simulink model "Aircraft_Power_Network"  (R2020a)
settings: Solver=ode23t  StartTime=0.0  StopTime=40  RelTol=1e-3  EnableMultiTasking=on
PostLoadFcn:
  | %load PQ_DATA4
  | Flight_Cycle_Num = 1;
  | 
  | warning off Simulink:blocks:MatchingFromNotFound
  | warning off Simulink:blocks:MatchingGotoNotFound
  | warning off Simulink:Engine:SaveWithParameterizedLinks_Warning
  | warning off MATLAB:nearlySingularMatrix
  | warning off simscape:compiler:sli:init:SolverNotRecommended
  | warning off Simulink:ID:DuplicateSID
  | warning off Simulink:Engine:UINotUpdatedDuringRapidAccelSim
  | warning off Simulink:SampleTime:IllegalIPortRateTrans
  | warning off Simulink:SampleTime:SourceInheritedTS
StartFcn:
  | tic;
StopFcn:
  | Elapsed_Sim_Time = toc; disp(['Elapsed time is ' num2str(Elapsed_Sim_Time)])
undefined symbols (not defined in the file or in its folder): Ts
libraries: powerlib x6, powerlib_meascontrol x4, Actuator_AC_Lib x2, Lamp_Lib x2, Pump_Lib x2, DC_Loads_Lib x2, Distribution_Lib x1, Generator_Lib x1, Power_Calc_Lib x1
Description:
  | Copyright 2014-2020 The MathWorks, Inc.
settings Model: TunableVars=Flight_Cycle_Num  TunableVarsStorageClass=Auto  Creator=smiller  LastModifiedBy=smiller
settings DataIOCC: LimitDataPoints=on  SaveFormat=Array  ReturnWorkspaceOutputs=off
settings OptimizationCC: DefaultParameterBehavior=Inlined  OptimizeBlockIOStorage=off  BufferReuse=off  GlobalBufferReuse=off  ExpressionFolding=off  LocalBlockOutputs=off  LifeSpan=inf  OptimizeDataStoreBuffers=off  BusAssignmentInplaceUpdate=off
settings DebuggingCC: UnderspecifiedInitializationDetection=Classic  MergeDetectMultiDrivingBlocksExec=none  SolverPrmCheckMsg=warning  MultiTaskRateTransMsg=warning  AllowSymbolicDim=off  StateNameClashWarn=warning  PregeneratedLibrarySubsystemCodeDiagnostic=none  SFUnexpectedBacktrackingDiag=warning  SFNoUnconditionalDefaultTransitionDiag=warning  SFExecutionAtInitializationDiag=none  ArithmeticOperatorsInVariantConditions=warning
settings HardwareCC: ProdBitPerPointer=32  ProdBitPerSizeT=32  ProdBitPerPtrDiffT=32  ProdLargestAtomicFloat=None  ProdIntDivRoundTo=Undefined  ProdEndianess=Unspecified  ProdWordSize=32  ProdHWDeviceType=32-bit Generic
settings ModelReferenceCC: PropagateSignalLabelsOutOfModel=off
settings SFSimCC: SimUseLocalCustomCode=off  CustomCodeUndefinedFunction=UseInterfaceOnly
settings RTWCC: RTWUseLocalCustomCode=off
settings CodeAppCC: StateflowObjectComments=on
settings GRTTargetCC: TargetLangStandard=C89/C90 (ANSI)  CombineOutputUpdateFcns=off  GRTInterface=on
settings ConfigComp: CovMetricSettings=dw  CovHtmlReporting=on  CovSaveCumulativeToWorkspaceVar=on  CovSaveSingleToWorkspaceVar=on  CovExternalEMLEnable=off  CovSFcnEnable=off
settings SimscapeCC: SimscapeNormalizeSystem=off

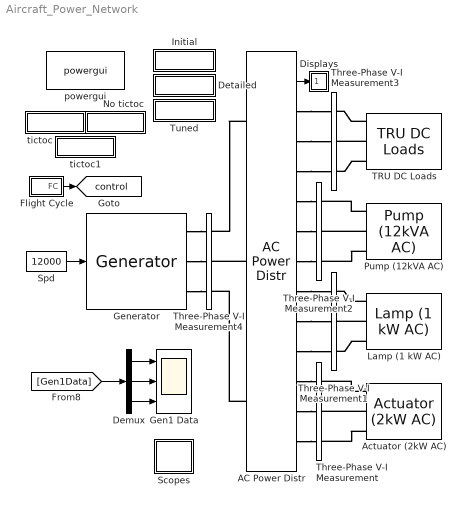
== system Aircraft_Power_Network ==
  AC Power Distr : Distribution_Lib/AC Power Distr  LabelModeActiveChoice=Phasor  ModelType=Phasor
      settings: AttributesFormatString=%<BlockChoice>
  Actuator (2kW AC) : Actuator_AC_Lib/Actuator (2kW AC)  LabelModeActiveChoice=Phasor  ModelType=Phasor  PQ_Model=Tuned
      link override Detailed/PM Synchronous Motor Drive/Output Bus Selector: OutputSignals=Rotor speed wm (rad/s)
      link override Detailed/PM Synchronous Motor Drive/Permanent Magnet Synchronous Machine: MechanicalLoad=Torque Tm  VoltageCst=126.966  TorqueCst=1.05
      link override Detailed/PM Synchronous Motor Drive/VECT: modulationType=Hysteresis  Ts_vect=20e-6  h=0.1  freq_max=20e3  fc_bus=50  car_freq=20000  nb_p=4  machineConstant=Flux linkage established by magnets (V.s)  fluxConstant=0.175  voltageConstant=126.966  torqueConstant=1.05  kp_Id=200  ki_Id=1000  kp_Iq=200  ki_Iq=1000
      link override Detailed/PM Synchronous Motor Drive1/VECT: freq_max=20e3  Ts_vect=50e-6  h=0.1  nb_p=4  lambda=0.175
      link override Phasor/Calc PQ: BlockChoice=Initial
      settings: AttributesFormatString=%<BlockChoice>
  Demux : Demux  Outputs=[2 1 1]
  Detailed : Subsystem
      settings: OpenFcn=Select_APN_Model_Config(bdroot,'Detailed');
      mask Display: disp('Detailed');
  Displays : Subsystem
      mask Display: disp('D')
  Flight Cycle : Subsystem
      mask Display: disp(num2str(evalin('base','Flight_Cycle_Num')));
  Gen1 Data : Scope  NumInputPorts=3
  Generator : Generator_Lib/Generator  LabelModeActiveChoice=Ideal  GenType=Ideal  GenTypeDCLink=Ideal
      link override VSCF DC Link/DC Link Gen: BlockChoice=Ideal
      link override VSCF DC Link/DC Link Gen/Sync Mach/Simplified Synchronous Machine SI Units/Electrical model: BlockChoice=Phasor
      link override VSCF DC Link/DC Link Gen/Sync Mach/Simplified Synchronous Machine SI Units/From: GotoTag=tp2df5cfb3_b42e_4dd4_aed6_ebb45f5ee09b
      link override VSCF DC Link/DC Link Gen/Sync Mach/Simplified Synchronous Machine SI Units/Goto: GotoTag=tp9f3ab3a0_63ac_4acf_b3bd_c670964be41e
      link override VSCF DC Link/DC Link Gen/Sync Mach/Simplified Synchronous Machine SI Units/Mechanical model: BlockChoice=Phasor w input
      settings: AttributesFormatString=%<BlockChoice>
  Initial : Subsystem
      settings: OpenFcn=Select_APN_Model_Config(bdroot,'Initial');
      mask Display: disp('Initial');
  Lamp (1 kW AC) : Lamp_Lib/Lamp (1 kW AC)  RequirementInfo={} %GIDa_b4ebd6a2_cdd2_4eca_9ae5_96943b3eee14  LabelModeActiveChoice=Phasor  ModelType=Phasor  PQ_Model=Tuned
      link override Phasor/Calc PQ: BlockChoice=Initial
      settings: AttributesFormatString=%<BlockChoice>
  No tictoc : Subsystem
      settings: OpenFcn=|
      | set_param(bdroot,'StartFcn','');
      | set_param(bdroot,'StopFcn','');
      mask Display: disp('No tictoc')
  Pump (12kVA AC) : Pump_Lib/Pump (12kVA AC)  LabelModeActiveChoice=Phasor  ModelType=Phasor  PQ_Model=Tuned
      link override Phasor/Calc PQ: BlockChoice=Initial
      settings: AttributesFormatString=%<BlockChoice>
  Scopes : Subsystem
  Spd : Constant  Value=12000
  TRU DC Loads : DC_Loads_Lib/TRU DC Loads  RequirementInfo={} %GIDa_0f590c74_ec2b_4e2c_b0ce_7c36d608bdaa  LabelModeActiveChoice=Phasor  ModelType=Phasor  PQ_Model=Tuned
      link override Phasor/Calc PQ: BlockChoice=Initial
      settings: AttributesFormatString=%<BlockChoice>
  Three-Phase V-I Measurement : powerlib/Measurements/Three-Phase V-I Measurement  VoltageMeasurement=phase-to-ground  SetLabelV=on  LabelV=Vabc_BDMotor  Vpu=off  VpuLL=off  CurrentMeasurement=yes  SetLabelI=on  LabelI=Iabc_BDMotor  Ipu=off  Pbase=100e6  Vbase=500e3  OutputType=Magnitude  PhasorSimulation=on  PSBequivalent=0
  Three-Phase V-I Measurement1 : powerlib/Measurements/Three-Phase V-I Measurement  VoltageMeasurement=phase-to-ground  SetLabelV=on  LabelV=Vabc_Lamp  Vpu=off  VpuLL=off  CurrentMeasurement=yes  SetLabelI=on  LabelI=Iabc_Lamp  Ipu=off  Pbase=100e6  Vbase=500e3  OutputType=Magnitude  PhasorSimulation=on  PSBequivalent=0
  Three-Phase V-I Measurement2 : powerlib/Measurements/Three-Phase V-I Measurement  VoltageMeasurement=phase-to-ground  SetLabelV=on  LabelV=Vabc_InductionMotor  Vpu=off  VpuLL=off  CurrentMeasurement=yes  SetLabelI=on  LabelI=Iabc_InductionMotor  Ipu=off  Pbase=100e6  Vbase=500e3  OutputType=Magnitude  PhasorSimulation=on  PSBequivalent=0
  Three-Phase V-I Measurement3 : powerlib/Measurements/Three-Phase V-I Measurement  VoltageMeasurement=phase-to-ground  SetLabelV=on  LabelV=Vabc_TRU  Vpu=off  VpuLL=off  CurrentMeasurement=yes  SetLabelI=on  LabelI=Iabc_TRU  Ipu=off  Pbase=100e6  Vbase=500e3  OutputType=Magnitude  PhasorSimulation=on  PSBequivalent=0
  Three-Phase V-I Measurement4 : powerlib/Measurements/Three-Phase V-I Measurement  VoltageMeasurement=phase-to-ground  SetLabelV=on  LabelV=Vabc_GEN  Vpu=off  VpuLL=off  CurrentMeasurement=yes  SetLabelI=on  LabelI=Iabc_GEN  Ipu=off  Pbase=100e6  Vbase=500e3  OutputType=Magnitude  PhasorSimulation=on  PSBequivalent=0
  Tuned : Subsystem
      settings: OpenFcn=Select_APN_Model_Config(bdroot,'Tuned');
      mask Display: disp('Tuned');
  powergui : powerlib/powergui  SimulationMode=Phasor  SampleTime=Ts  frequency=400  Iterations=50  frequencyindice=400  Pbase=100e6  ErrMax=0.0001  UnitsV=kV  UnitsW=MW  buscounter=0  FunctionMessages=off  echomessages=off  EnableUseOfTLC=off  CurrentSourceSwitches=off  DisableSnubberDevices=off  DisableRonSwitches=off  DisableVfSwitches=off  DisplayEquations=off  AutomaticDiscreteSolvers=off  SolverType=Tustin  Interpol=off  ExternalGateDelay=off  methode=off  Ts=0  x0status=blocks  SPID=off  SwTol=0  HookPort=off  NonlinearTolerance=0  nMaxIteration=15  ContinueOnMaxIteration=off  RestoreLinks=no  ResistiveCurrentMeasurement=off  Frange=[0:2:500]  Ylog=off  Xlog=on  ShowGrid=off  save=off  variable=ZData  structure=Gen1_Vab  ZoomFFT=on  StartTime=0.3  cycles=1  DisplayStyle=1  fundamental=400  FreqAxis=on  MaxFrequency=8000  frequencyindicesteady=1  RmsSteady=1  display=off
  tictoc : Subsystem
      settings: OpenFcn=|
      | set_param(bdroot,'StartFcn','tic;');
      | set_param(bdroot,'StopFcn','Elapsed_Sim_Time = toc; disp([''Elapsed time is '' num2str(Elapsed_Sim_Time)])');
      mask Display: disp('tictoc')
  tictoc1 : Subsystem
      settings: OpenFcn=open('APN_Demo_Script.html')
      mask Display: disp('Script')
  tag scope: control=global
  wires:
  Flight Cycle/1(FC) -> [control]
  AC Power Distr/1 -> Displays/1(In1)
  Spd/1 -> Generator/1
  [Gen1Data] -> Demux/1
  Demux/1 -> Gen1 Data/1
  Demux/2 -> Gen1 Data/2
  Demux/3 -> Gen1 Data/3
  connections:
  Generator/RConn1 -- Three-Phase V-I Measurement4/LConn1
  Generator/RConn2 -- Three-Phase V-I Measurement4/LConn2
  Generator/RConn3 -- Three-Phase V-I Measurement4/LConn3
  AC Power Distr/LConn2 -- Three-Phase V-I Measurement4/RConn2
  Lamp (1 kW AC)/LConn3 -- Three-Phase V-I Measurement1/RConn3
  Actuator (2kW AC)/LConn2 -- Three-Phase V-I Measurement/RConn2
  AC Power Distr/RConn3 -- Three-Phase V-I Measurement3/LConn3
  AC Power Distr/RConn6 -- Three-Phase V-I Measurement2/LConn3
  Pump (12kVA AC)/LConn2 -- Three-Phase V-I Measurement2/RConn2
  TRU DC Loads/LConn3 -- Three-Phase V-I Measurement3/RConn3
  Actuator (2kW AC)/LConn3 -- Three-Phase V-I Measurement/RConn3
  Pump (12kVA AC)/LConn3 -- Three-Phase V-I Measurement2/RConn3
  AC Power Distr/RConn4 -- Three-Phase V-I Measurement2/LConn1
  TRU DC Loads/LConn1 -- Three-Phase V-I Measurement3/RConn1
  AC Power Distr/RConn11 -- Three-Phase V-I Measurement/LConn2
  Actuator (2kW AC)/LConn1 -- Three-Phase V-I Measurement/RConn1
  AC Power Distr/RConn8 -- Three-Phase V-I Measurement1/LConn2
  AC Power Distr/LConn3 -- Three-Phase V-I Measurement4/RConn3
  AC Power Distr/LConn1 -- Three-Phase V-I Measurement4/RConn1
  AC Power Distr/RConn12 -- Three-Phase V-I Measurement/LConn3
  AC Power Distr/RConn1 -- Three-Phase V-I Measurement3/LConn1
  AC Power Distr/RConn5 -- Three-Phase V-I Measurement2/LConn2
  AC Power Distr/RConn9 -- Three-Phase V-I Measurement1/LConn3
  TRU DC Loads/LConn2 -- Three-Phase V-I Measurement3/RConn2
  AC Power Distr/RConn7 -- Three-Phase V-I Measurement1/LConn1
  Lamp (1 kW AC)/LConn2 -- Three-Phase V-I Measurement1/RConn2
  AC Power Distr/RConn10 -- Three-Phase V-I Measurement/LConn1
  Lamp (1 kW AC)/LConn1 -- Three-Phase V-I Measurement1/RConn1
  AC Power Distr/RConn2 -- Three-Phase V-I Measurement3/LConn2
  Pump (12kVA AC)/LConn1 -- Three-Phase V-I Measurement2/RConn1

== system Aircraft_Power_Network/Detailed ==

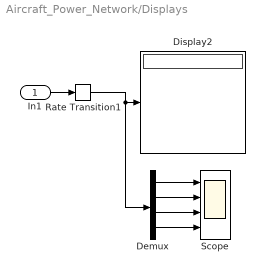
== system Aircraft_Power_Network/Displays ==
  In1 : Inport
  Demux : Demux
  Display2 : Display
      settings: Decimation=100  SampleTime=1e-2
  Rate Transition1 : RateTransition  OutPortSampleTimeOpt=Inherit  OutPortSampleTime=Ts
  Scope : Scope  NumInputPorts=4
  wires:
  In1/1 -> Rate Transition1/1
  Rate Transition1/1 -> Demux/1, Display2/1
  Demux/3 -> Scope/3
  Demux/4 -> Scope/4
  Demux/1 -> Scope/1
  Demux/2 -> Scope/2

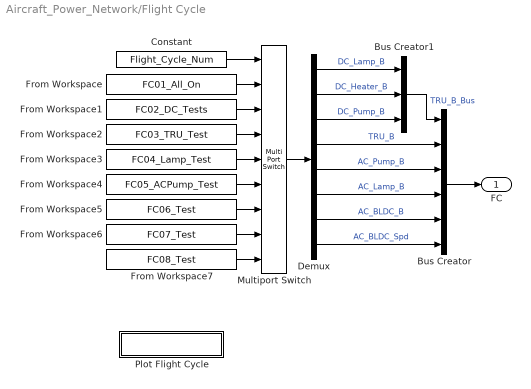
== system Aircraft_Power_Network/Flight Cycle ==
  Bus Creator : BusCreator  Inputs=6
  Bus Creator1 : BusCreator  Inputs=3
  Constant : Constant  Value=Flight_Cycle_Num
  Demux : Demux  Outputs=8
  From Workspace : FromWorkspace  VariableName=FC01_All_On  OutputAfterFinalValue=Holding final value
  From Workspace1 : FromWorkspace  VariableName=FC02_DC_Tests
  From Workspace2 : FromWorkspace  VariableName=FC03_TRU_Test
  From Workspace3 : FromWorkspace  VariableName=FC04_Lamp_Test
  From Workspace4 : FromWorkspace  VariableName=FC05_ACPump_Test  OutputAfterFinalValue=Holding final value
  From Workspace5 : FromWorkspace  VariableName=FC06_Test  OutputAfterFinalValue=Holding final value
  From Workspace6 : FromWorkspace  VariableName=FC07_Test  OutputAfterFinalValue=Holding final value
  From Workspace7 : FromWorkspace  VariableName=FC08_Test  OutputAfterFinalValue=Holding final value
  Multiport Switch : MultiPortSwitch  Inputs=8
  Plot Flight Cycle : Subsystem
      settings: OpenFcn=Plot_FC
      mask Display: disp('Plot Flight Cycle');
  FC : Outport  VectorParamsAs1DForOutWhenUnconnected=off
  wires:
  Bus Creator/1 -> FC/1
  Bus Creator1/1 -> Bus Creator/1  "TRU_B_Bus"
  From Workspace/1 -> Multiport Switch/2
  From Workspace1/1 -> Multiport Switch/3
  From Workspace2/1 -> Multiport Switch/4
  From Workspace3/1 -> Multiport Switch/5
  From Workspace4/1 -> Multiport Switch/6
  Multiport Switch/1 -> Demux/1
  Constant/1 -> Multiport Switch/1
  Demux/1 -> Bus Creator1/1  "DC_Lamp_B"
  Demux/2 -> Bus Creator1/2  "DC_Heater_B"
  Demux/3 -> Bus Creator1/3  "DC_Pump_B"
  Demux/4 -> Bus Creator/2  "TRU_B"
  Demux/5 -> Bus Creator/3  "AC_Pump_B"
  Demux/6 -> Bus Creator/4  "AC_Lamp_B"
  Demux/7 -> Bus Creator/5  "AC_BLDC_B"
  Demux/8 -> Bus Creator/6  "AC_BLDC_Spd"
  From Workspace5/1 -> Multiport Switch/7
  From Workspace6/1 -> Multiport Switch/8
  From Workspace7/1 -> Multiport Switch/9

== system Aircraft_Power_Network/Initial ==

== system Aircraft_Power_Network/No tictoc ==

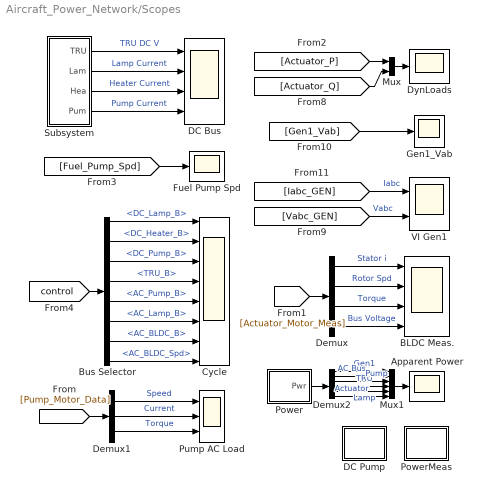
== system Aircraft_Power_Network/Scopes ==
  Apparent Power : Scope
  BLDC Meas. : Scope  NumInputPorts=4
  Bus Selector : BusSelector  OutputSignals=TRU_B_Bus.DC_Lamp_B,TRU_B_Bus.DC_Heater_B,TRU_B_Bus.DC_Pump_B,TRU_B,AC_Pump_B,AC_Lamp_B,AC_BLDC_B,AC_BLDC_Spd
  Cycle : Scope  NumInputPorts=8
  DC Bus : Scope  NumInputPorts=4
  DC Pump : Subsystem
  Demux : Demux  Outputs=[1 2 2 1]
  Demux1 : Demux  Outputs=3
  Demux2 : Demux  Outputs=6
  DynLoads : Scope
  Fuel Pump Spd : Scope
  Gen1_Vab : Scope
  Mux : Mux  Inputs=2
  Mux1 : Mux  Inputs=6
  Power : Subsystem
  PowerMeas : Subsystem
  Pump AC Load : Scope  NumInputPorts=3
  Subsystem : Subsystem
  VI Gen1 : Scope  NumInputPorts=2
  wires:
  [Fuel_Pump_Spd] -> Fuel Pump Spd/1
  Demux/1 -> BLDC Meas./1  "Stator i"
  Demux/2 -> BLDC Meas./2  "Rotor Spd"
  Demux/3 -> BLDC Meas./3  "Torque"
  Demux/4 -> BLDC Meas./4  "Bus Voltage"
  [Actuator_Motor_Meas] -> Demux/1
  Subsystem/2(Lam) -> DC Bus/2  "Lamp Current"
  Subsystem/3(Hea) -> DC Bus/3  "Heater Current"
  Subsystem/4(Pum) -> DC Bus/4  "Pump Current"
  Subsystem/1(TRU) -> DC Bus/1  "TRU DC V"
  [Gen1_Vab] -> Gen1_Vab/1
  [control] -> Bus Selector/1
  Bus Selector/8 -> Cycle/8  "<AC_BLDC_Spd>"
  Bus Selector/7 -> Cycle/7  "<AC_BLDC_B>"
  Bus Selector/5 -> Cycle/5  "<AC_Pump_B>"
  Bus Selector/6 -> Cycle/6  "<AC_Lamp_B>"
  Bus Selector/1 -> Cycle/1  "<DC_Lamp_B>"
  Bus Selector/2 -> Cycle/2  "<DC_Heater_B>"
  Bus Selector/4 -> Cycle/4  "<TRU_B>"
  Bus Selector/3 -> Cycle/3  "<DC_Pump_B>"
  [Actuator_P] -> Mux/1
  Mux/1 -> DynLoads/1
  [Actuator_Q] -> Mux/2
  [Iabc_GEN] -> VI Gen1/1  "Iabc"
  [Vabc_GEN] -> VI Gen1/2  "Vabc"
  Power/1(Pwr) -> Demux2/1
  Demux1/3 -> Pump AC Load/3  "Torque"
  Demux1/1 -> Pump AC Load/1  "Speed"
  Demux1/2 -> Pump AC Load/2  "Current"
  [Pump_Motor_Data] -> Demux1/1
  Demux2/6 -> Mux1/6  "Actuator"
  Demux2/1 -> Mux1/1  "Gen1"
  Demux2/2 -> Mux1/2  "AC Bus"
  Demux2/4 -> Mux1/4  "TRU"
  Demux2/3 -> Mux1/3  "Pump"
  Demux2/5 -> Mux1/5  "Lamp"
  Mux1/1 -> Apparent Power/1

== system Aircraft_Power_Network/Tuned ==

== system Aircraft_Power_Network/tictoc ==

== system Aircraft_Power_Network/tictoc1 ==

== system Aircraft_Power_Network/Flight Cycle/Plot Flight Cycle ==

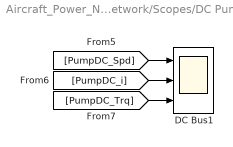
== system Aircraft_Power_Network/Scopes/DC Pump ==
  DC Bus1 : Scope  NumInputPorts=3
  wires:
  [PumpDC_i] -> DC Bus1/2
  [PumpDC_Spd] -> DC Bus1/1
  [PumpDC_Trq] -> DC Bus1/3

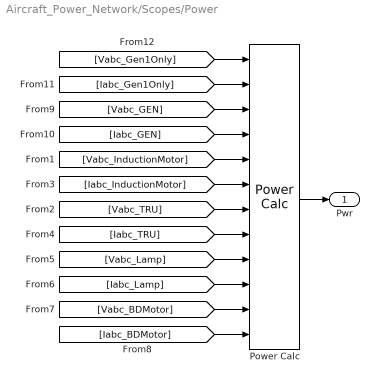
== system Aircraft_Power_Network/Scopes/Power ==
  Power Calc : Power_Calc_Lib/Power Calc  LabelModeActiveChoice=Phasor  ModelType=Phasor
      settings: AttributesFormatString=%<BlockChoice>
  Pwr : Outport  VectorParamsAs1DForOutWhenUnconnected=off
  wires:
  [Vabc_Gen1Only] -> Power Calc/1
  [Iabc_Gen1Only] -> Power Calc/2
  [Vabc_GEN] -> Power Calc/3
  [Iabc_GEN] -> Power Calc/4
  [Vabc_InductionMotor] -> Power Calc/5
  [Iabc_InductionMotor] -> Power Calc/6
  [Vabc_TRU] -> Power Calc/7
  [Iabc_TRU] -> Power Calc/8
  [Vabc_Lamp] -> Power Calc/9
  [Iabc_Lamp] -> Power Calc/10
  Power Calc/1 -> Pwr/1
  [Vabc_BDMotor] -> Power Calc/11
  [Iabc_BDMotor] -> Power Calc/12

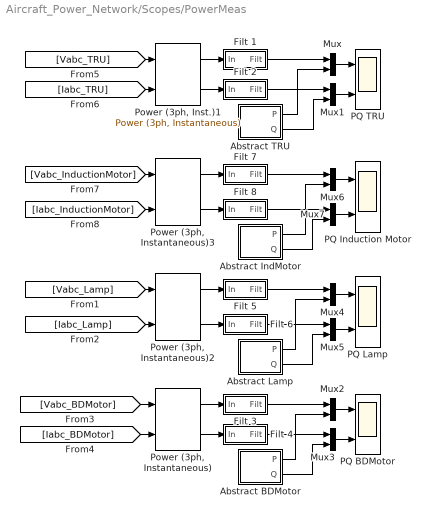
== system Aircraft_Power_Network/Scopes/PowerMeas ==
  Abstract BDMotor : Subsystem
  Abstract IndMotor : Subsystem
  Abstract Lamp : Subsystem
  Abstract TRU : Subsystem
  Filt 1 : Subsystem
  Filt 2 : Subsystem
  Filt 3 : Subsystem
  Filt 4 : Subsystem
  Filt 5 : Subsystem
  Filt 6 : Subsystem
  Filt 7 : Subsystem
  Filt 8 : Subsystem
  Mux{,1..7} (8 alike) : Mux  Inputs=2
  PQ BDMotor : Scope  NumInputPorts=2
  PQ Induction Motor : Scope  NumInputPorts=2
  PQ Lamp : Scope  NumInputPorts=2
  PQ TRU : Scope  NumInputPorts=2
  "Power (3ph, Instantaneous)" : powerlib_meascontrol/Measurements/Power (3ph, Instantaneous)
  "Power (3ph, Instantaneous)2" : powerlib_meascontrol/Measurements/Power (3ph, Instantaneous)
  "Power (3ph, Instantaneous)3" : powerlib_meascontrol/Measurements/Power (3ph, Instantaneous)
  "Power (3ph, Inst.)1" : powerlib_meascontrol/Measurements/Power (3ph, Instantaneous)
  wires:
  Filt 3/1(Filt) -> Mux2/1
  [Vabc_BDMotor] -> "Power (3ph, Instantaneous)"/1
  [Iabc_TRU] -> "Power (3ph, Inst.)1"/2
  Filt 1/1(Filt) -> Mux/1
  "Power (3ph, Inst.)1"/2 -> Filt 2/1(In)
  "Power (3ph, Instantaneous)"/1 -> Filt 3/1(In)
  [Iabc_BDMotor] -> "Power (3ph, Instantaneous)"/2
  "Power (3ph, Instantaneous)"/2 -> Filt 4/1(In)
  Filt 2/1(Filt) -> Mux1/1
  [Vabc_TRU] -> "Power (3ph, Inst.)1"/1
  "Power (3ph, Inst.)1"/1 -> Filt 1/1(In)
  Filt 4/1(Filt) -> Mux3/1
  [Iabc_Lamp] -> "Power (3ph, Instantaneous)2"/2
  "Power (3ph, Instantaneous)2"/2 -> Filt 6/1(In)
  [Vabc_Lamp] -> "Power (3ph, Instantaneous)2"/1
  "Power (3ph, Instantaneous)2"/1 -> Filt 5/1(In)
  [Iabc_InductionMotor] -> "Power (3ph, Instantaneous)3"/2
  Filt 7/1(Filt) -> Mux6/1
  "Power (3ph, Instantaneous)3"/2 -> Filt 8/1(In)
  Filt 8/1(Filt) -> Mux7/1
  [Vabc_InductionMotor] -> "Power (3ph, Instantaneous)3"/1
  "Power (3ph, Instantaneous)3"/1 -> Filt 7/1(In)
  Mux/1 -> PQ TRU/1
  Mux1/1 -> PQ TRU/2
  Mux2/1 -> PQ BDMotor/1
  Mux3/1 -> PQ BDMotor/2
  Filt 5/1(Filt) -> Mux4/1
  Filt 6/1(Filt) -> Mux5/1
  Mux4/1 -> PQ Lamp/1
  Mux5/1 -> PQ Lamp/2
  Abstract TRU/1(P) -> Mux/2
  Abstract TRU/2(Q) -> Mux1/2
  Abstract BDMotor/1(P) -> Mux2/2
  Abstract BDMotor/2(Q) -> Mux3/2
  Abstract Lamp/1(P) -> Mux4/2
  Abstract Lamp/2(Q) -> Mux5/2
  Mux6/1 -> PQ Induction Motor/1
  Mux7/1 -> PQ Induction Motor/2
  Abstract IndMotor/1(P) -> Mux6/2
  Abstract IndMotor/2(Q) -> Mux7/2

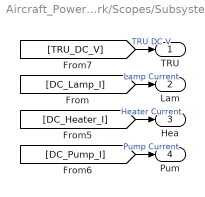
== system Aircraft_Power_Network/Scopes/Subsystem ==
  TRU : Outport  VectorParamsAs1DForOutWhenUnconnected=off
  Lam : Outport  Port=2  VectorParamsAs1DForOutWhenUnconnected=off
  Hea : Outport  Port=3  VectorParamsAs1DForOutWhenUnconnected=off
  Pum : Outport  Port=4  VectorParamsAs1DForOutWhenUnconnected=off
  wires:
  [DC_Lamp_I] -> Lam/1  "Lamp Current"
  [DC_Pump_I] -> Pum/1  "Pump Current"
  [DC_Heater_I] -> Hea/1  "Heater Current"
  [TRU_DC_V] -> TRU/1  "TRU DC V"

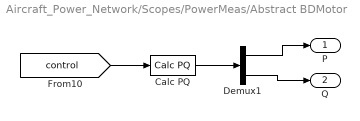
== system Aircraft_Power_Network/Scopes/PowerMeas/Abstract BDMotor ==
  Calc PQ : Actuator_AC_Lib/Actuator (2kW AC)/Phasor/Calc PQ  LabelModeActiveChoice=Initial  PQ_Model=Initial
      settings: AttributesFormatString=%<LabelModeActiveChoice>
  Demux1 : Demux  Outputs=2
  P : Outport  VectorParamsAs1DForOutWhenUnconnected=off
  Q : Outport  Port=2  VectorParamsAs1DForOutWhenUnconnected=off
  wires:
  [control] -> Calc PQ/1
  Calc PQ/1 -> Demux1/1
  Demux1/1 -> P/1
  Demux1/2 -> Q/1

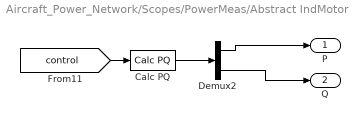
== system Aircraft_Power_Network/Scopes/PowerMeas/Abstract IndMotor ==
  Calc PQ : Pump_Lib/Pump (12kVA AC)/Phasor/Calc PQ  LabelModeActiveChoice=Initial  PQ_Model=Initial
      settings: AttributesFormatString=%<BlockChoice>
  Demux2 : Demux  Outputs=2
  P : Outport  VectorParamsAs1DForOutWhenUnconnected=off
  Q : Outport  Port=2  VectorParamsAs1DForOutWhenUnconnected=off
  wires:
  Calc PQ/1 -> Demux2/1
  Demux2/2 -> Q/1
  Demux2/1 -> P/1
  [control] -> Calc PQ/1

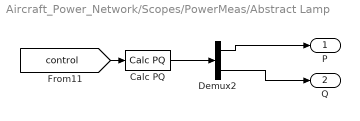
== system Aircraft_Power_Network/Scopes/PowerMeas/Abstract Lamp ==
  Calc PQ : Lamp_Lib/Lamp (1 kW AC)/Phasor/Calc PQ  LabelModeActiveChoice=Initial  PQ_Model=Initial
      settings: AttributesFormatString=%<LabelModeActiveChoice>
  Demux2 : Demux  Outputs=2
  P : Outport  VectorParamsAs1DForOutWhenUnconnected=off
  Q : Outport  Port=2  VectorParamsAs1DForOutWhenUnconnected=off
  wires:
  [control] -> Calc PQ/1
  Demux2/1 -> P/1
  Demux2/2 -> Q/1
  Calc PQ/1 -> Demux2/1

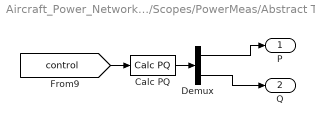
== system Aircraft_Power_Network/Scopes/PowerMeas/Abstract TRU ==
  Calc PQ : DC_Loads_Lib/TRU DC Loads/Phasor/Calc PQ  LabelModeActiveChoice=Initial  PQ_Model=Initial
      settings: AttributesFormatString=%<LabelModeActiveChoice>
  Demux : Demux  Outputs=2
  P : Outport  VectorParamsAs1DForOutWhenUnconnected=off
  Q : Outport  Port=2  VectorParamsAs1DForOutWhenUnconnected=off
  wires:
  [control] -> Calc PQ/1
  Calc PQ/1 -> Demux/1
  Demux/1 -> P/1
  Demux/2 -> Q/1

== system Aircraft_Power_Network/Scopes/PowerMeas/Filt 1 ==
  In : Inport
  Mux : Mux  Inputs=2
  Transfer Fcn : TransferFcn  Denominator=[0.01 1]
  Filt : Outport  VectorParamsAs1DForOutWhenUnconnected=off
  wires:
  Transfer Fcn/1 -> Mux/2
  In/1 -> Transfer Fcn/1, Mux/1
  Mux/1 -> Filt/1

== system Aircraft_Power_Network/Scopes/PowerMeas/Filt 2 ==
  In : Inport
  Mux : Mux  Inputs=2
  Transfer Fcn : TransferFcn  Denominator=[0.01 1]
  Filt : Outport  VectorParamsAs1DForOutWhenUnconnected=off
  wires:
  Mux/1 -> Filt/1
  In/1 -> Mux/1, Transfer Fcn/1
  Transfer Fcn/1 -> Mux/2

== system Aircraft_Power_Network/Scopes/PowerMeas/Filt 3 ==
  In : Inport
  Mux : Mux  Inputs=2
  Transfer Fcn : TransferFcn  Denominator=[0.01 1]
  Filt : Outport  VectorParamsAs1DForOutWhenUnconnected=off
  wires:
  Transfer Fcn/1 -> Mux/2
  In/1 -> Transfer Fcn/1, Mux/1
  Mux/1 -> Filt/1

== system Aircraft_Power_Network/Scopes/PowerMeas/Filt 4 ==
  In : Inport
  Mux : Mux  Inputs=2
  Transfer Fcn : TransferFcn  Denominator=[0.01 1]
  Filt : Outport  VectorParamsAs1DForOutWhenUnconnected=off
  wires:
  Mux/1 -> Filt/1
  In/1 -> Mux/1, Transfer Fcn/1
  Transfer Fcn/1 -> Mux/2

== system Aircraft_Power_Network/Scopes/PowerMeas/Filt 5 ==
  In : Inport
  Mux : Mux  Inputs=2
  Transfer Fcn : TransferFcn  Denominator=[0.01 1]
  Filt : Outport  VectorParamsAs1DForOutWhenUnconnected=off
  wires:
  Transfer Fcn/1 -> Mux/2
  In/1 -> Transfer Fcn/1, Mux/1
  Mux/1 -> Filt/1

== system Aircraft_Power_Network/Scopes/PowerMeas/Filt 6 ==
  In : Inport
  Mux : Mux  Inputs=2
  Transfer Fcn : TransferFcn  Denominator=[0.01 1]
  Filt : Outport  VectorParamsAs1DForOutWhenUnconnected=off
  wires:
  Mux/1 -> Filt/1
  In/1 -> Mux/1, Transfer Fcn/1
  Transfer Fcn/1 -> Mux/2

== system Aircraft_Power_Network/Scopes/PowerMeas/Filt 7 ==
  In : Inport
  Mux : Mux  Inputs=2
  Transfer Fcn : TransferFcn  Denominator=[0.01 1]
  Filt : Outport  VectorParamsAs1DForOutWhenUnconnected=off
  wires:
  Transfer Fcn/1 -> Mux/2
  In/1 -> Transfer Fcn/1, Mux/1
  Mux/1 -> Filt/1

== system Aircraft_Power_Network/Scopes/PowerMeas/Filt 8 ==
  In : Inport
  Mux : Mux  Inputs=2
  Transfer Fcn : TransferFcn  Denominator=[0.01 1]
  Filt : Outport  VectorParamsAs1DForOutWhenUnconnected=off
  wires:
  Mux/1 -> Filt/1
  In/1 -> Mux/1, Transfer Fcn/1
  Transfer Fcn/1 -> Mux/2
